simulink model "Arm_Mobile_Simulation_MATLAB24"  (R2024b)
settings: Solver=ode23t  StartTime=0.0  StopTime=25  MaxStep=dt  RelTol=1e-3
InitFcn:
  | dt = 0.01;
  | 
  | OP = 1;
  | 
  | %% Contact Data
  | G_K = 1e6;
  | G_B = 1e3;
  | 
  | G_Mu_s = 0.3;
  | G_Mu_k = 0.5;
  | 
  | %% Object Position for Pick and Drop
  | 
  | PL = [1.2 0 0.675];  % Pick location
  | 
  | PD = [1.4 0.8 0.475]; % Drop location
  | 
  | 
  | %% SimData
  | % Simscape(TM) Multibody(TM) version: 7.4
  | 
  | % This is a model data file derived from a Simscape Multibody Import XML file using the smimport function.
  | % The data in this file sets the block parameter values in an imported Simscape Multibody model.
  | % For more information on this file, see the smimport function help page in the Simscape Multibody documentation.
  | % You can modify numerical values, but avoid any other changes to this file.
  | % Do not add code to this file. Do not edit the physical units shown in comments.
  | 
  | %%%VariableName:smiData
  | 
  | 
  | %============= RigidTransform =============%
  | 
  | 
  | %Initialize the RigidTransform structure array by filling in null values.
  | smiData.RigidTransform(13).translation = [0.0 0.0 0.0];
  | smiData.RigidTransform(13).angle = 0.0;
  | smiData.RigidTransform(13).axis = [0.0 0.0 0.0];
  | smiData.RigidTransform(13).ID = '';
  | 
  | %Translation Method - Cartesian
  | %Rotation Method - Arbitrary Axis
  | smiData.RigidTransform(1).translation = [112.76762317970824 466.03898900587342 544.6225551646221];  % mm
  | smiData.RigidTransform(1).angle = 2.0943951023931953;  % rad
  | smiData.RigidTransform(1).axis = [-0.57735026918962584 -0.57735026918962584 -0.57735026918962584];
  | smiData.RigidTransform(1).ID = 'B[J1-1:-:J2-1]';
  | 
  | %Translation Method - Cartesian
  | %Rotation Method - Arbitrary Axis
  | smiData.RigidTransform(2).translation = [112.76762317970881 466.03898900587347 544.62255516462187];  % mm
  | smiData.RigidTransform(2).angle = 2.0943951023931957;  % rad
  | smiData.RigidTransform(2).axis = [-0.57735026918962584 -0.57735026918962573 -0.57735026918962573];
  | smiData.RigidTransform(2).ID = 'F[J1-1:-:J2-1]';
  | 
  | %Translation Method - Cartesian
  | %Rotation Method - Arbitrary Axis
  | smiData.RigidTransform(3).translation = [122.68366911264206 748.03898900587353 274.20311793228069];  % mm
  | smiData.RigidTransform(3).angle = 2.2406646857653398;  % rad
  | smiData.RigidTransform(3).axis = [0.61891214827171492 0.61891214827171503 0.48362744488229914];
  | smiData.RigidTransform(3).ID = 'B[J2-1:-:J3-1]';
  | 
  | ... (+181 lines)
undefined symbols (not defined in the file): smiData, X, Y, Z
libraries: sm_lib x161, nesl_utility x26
(part 4 of 4)

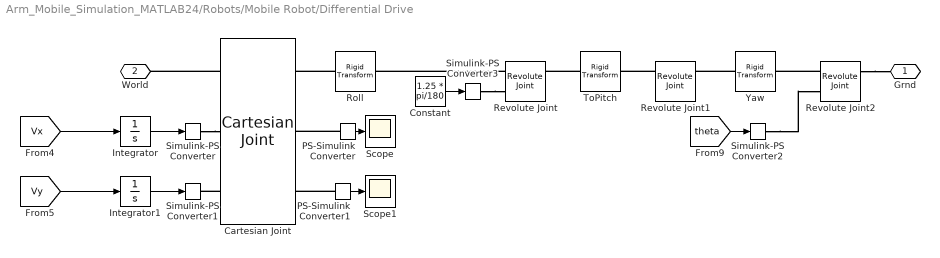
== system Arm_Mobile_Simulation_MATLAB24/Robots/Mobile Robot/Differential Drive ==
  Cartesian Joint : sm_lib/Joints/Cartesian Joint  JointMode=Normal  CompositeWrenchDir=FollowerOnBase  CompositeWrenchFrame=BaseFrame  SenseConstraintForce=off  SenseConstraintTorque=off  SenseTotalForce=off  SenseTotalTorque=off  PxPositionTargetSpecify=off  PxPositionTargetPriority=High  PxPositionTargetValue=0  PxPositionTargetValueUnits=m  PxVelocityTargetSpecify=off  PxVelocityTargetPriority=High  PxVelocityTargetValue=0  PxVelocityTargetValueUnits=m/s  PxEquilibriumPosition=0  PxEquilibriumPositionUnits=m  PxSpringStiffness=0  PxSpringStiffnessUnits=N/m  PxDampingCoefficient=0  PxDampingCoefficientUnits=N/(m/s)  PxLowerLimitSpecify=off  PxLowerLimitBound=-1  PxLowerLimitBoundUnits=m  PxLowerLimitStiffness=1e6  PxLowerLimitStiffnessUnits=N/m  PxLowerLimitDamping=1e3  PxLowerLimitDampingUnits=N/(m/s)  PxLowerLimitTransitionRegionWidth=1e-4  PxLowerLimitTransitionRegionWidthUnits=m  PxUpperLimitSpecify=off  PxUpperLimitBound=1  PxUpperLimitBoundUnits=m  PxUpperLimitStiffness=1e6  PxUpperLimitStiffnessUnits=N/m  PxUpperLimitDamping=1e3  PxUpperLimitDampingUnits=N/(m/s)  PxUpperLimitTransitionRegionWidth=1e-4  PxUpperLimitTransitionRegionWidthUnits=m  PxTorqueActuationMode=ComputedTorque  PxMotionActuationMode=InputMotion  PxSensePosition=on  PxSenseVelocity=off  PxSenseAcceleration=off  PxSenseTorqueForce=off  PxSenseLowerLimitTorqueForce=off  PxSenseUpperLimitTorqueForce=off  PyPositionTargetSpecify=off  PyPositionTargetPriority=High  PyPositionTargetValue=0  PyPositionTargetValueUnits=m  PyVelocityTargetSpecify=off  PyVelocityTargetPriority=High  PyVelocityTargetValue=0  PyVelocityTargetValueUnits=m/s  PyEquilibriumPosition=0  PyEquilibriumPositionUnits=m  PySpringStiffness=0  PySpringStiffnessUnits=N/m  PyDampingCoefficient=0  PyDampingCoefficientUnits=N/(m/s)  PyLowerLimitSpecify=off  PyLowerLimitBound=-1  PyLowerLimitBoundUnits=m  PyLowerLimitStiffness=1e6  PyLowerLimitStiffnessUnits=N/m  PyLowerLimitDamping=1e3  PyLowerLimitDampingUnits=N/(m/s)  PyLowerLimitTransitionRegionWidth=1e-4  PyLowerLimitTransitionRegionWidthUnits=m  PyUpperLimitSpecify=off  PyUpperLimitBound=1  PyUpperLimitBoundUnits=m  PyUpperLimitStiffness=1e6  PyUpperLimitStiffnessUnits=N/m  PyUpperLimitDamping=1e3  PyUpperLimitDampingUnits=N/(m/s)  PyUpperLimitTransitionRegionWidth=1e-4  PyUpperLimitTransitionRegionWidthUnits=m  PyTorqueActuationMode=ComputedTorque  PyMotionActuationMode=InputMotion  PySensePosition=on  PySenseVelocity=off  PySenseAcceleration=off  PySenseTorqueForce=off  PySenseLowerLimitTorqueForce=off  PySenseUpperLimitTorqueForce=off  PzPositionTargetSpecify=off  PzPositionTargetPriority=High  PzPositionTargetValue=0  PzPositionTargetValueUnits=m  PzVelocityTargetSpecify=off  PzVelocityTargetPriority=High  PzVelocityTargetValue=0  PzVelocityTargetValueUnits=m/s  PzEquilibriumPosition=0  PzEquilibriumPositionUnits=m  PzSpringStiffness=0  PzSpringStiffnessUnits=N/m  PzDampingCoefficient=0  PzDampingCoefficientUnits=N/(m/s)  PzLowerLimitSpecify=off  PzLowerLimitBound=-1  PzLowerLimitBoundUnits=m  PzLowerLimitStiffness=1e6  PzLowerLimitStiffnessUnits=N/m  PzLowerLimitDamping=1e3  PzLowerLimitDampingUnits=N/(m/s)  PzLowerLimitTransitionRegionWidth=1e-4  PzLowerLimitTransitionRegionWidthUnits=m  PzUpperLimitSpecify=off  PzUpperLimitBound=1  PzUpperLimitBoundUnits=m  PzUpperLimitStiffness=1e6  PzUpperLimitStiffnessUnits=N/m  PzUpperLimitDamping=1e3  PzUpperLimitDampingUnits=N/(m/s)  PzUpperLimitTransitionRegionWidth=1e-4  PzUpperLimitTransitionRegionWidthUnits=m  PzTorqueActuationMode=NoTorque  PzMotionActuationMode=ComputedMotion  PzSensePosition=off  PzSenseVelocity=off  PzSenseAcceleration=off  PzSenseTorqueForce=off  PzSenseLowerLimitTorqueForce=off  PzSenseUpperLimitTorqueForce=off
  Constant : Constant  Value=1.25 * pi/180
  Integrator : Integrator
  Integrator1 : Integrator
  PS-Simulink Converter : nesl_utility/PS-Simulink Converter  PhysicalDomain=network_engine_domain  SubClassName=ps_output  LeftPortType=input  RightPortType=output  PseudoPeriodic=off  Frequencies=[]  VectorFormat=1-D array  Unit=inherit  AffineConversion=off
  PS-Simulink Converter1 : nesl_utility/PS-Simulink Converter  PhysicalDomain=network_engine_domain  SubClassName=ps_output  LeftPortType=input  RightPortType=output  PseudoPeriodic=off  Frequencies=[]  VectorFormat=1-D array  Unit=inherit  AffineConversion=off
  Revolute Joint : sm_lib/Joints/Revolute Joint  JointMode=Normal  CompositeWrenchDir=FollowerOnBase  CompositeWrenchFrame=BaseFrame  SenseConstraintForce=off  SenseConstraintTorque=off  SenseTotalForce=off  SenseTotalTorque=off  PositionTargetSpecify=off  PositionTargetPriority=High  PositionTargetValue=90  PositionTargetValueUnits=deg  VelocityTargetSpecify=off  VelocityTargetPriority=High  VelocityTargetValue=0  VelocityTargetValueUnits=deg/s  EquilibriumPosition=0  EquilibriumPositionUnits=deg  SpringStiffness=0  SpringStiffnessUnits=N*m/deg  DampingCoefficient=0  DampingCoefficientUnits=N*m/(deg/s)  LowerLimitSpecify=off  LowerLimitBound=-90  LowerLimitBoundUnits=deg  LowerLimitStiffness=1e4  LowerLimitStiffnessUnits=N*m/deg  LowerLimitDamping=10  LowerLimitDampingUnits=N*m/(deg/s)  LowerLimitTransitionRegionWidth=0.1  LowerLimitTransitionRegionWidthUnits=deg  UpperLimitSpecify=off  UpperLimitBound=90  UpperLimitBoundUnits=deg  UpperLimitStiffness=1e4  UpperLimitStiffnessUnits=N*m/deg  UpperLimitDamping=10  UpperLimitDampingUnits=N*m/(deg/s)  UpperLimitTransitionRegionWidth=0.1  UpperLimitTransitionRegionWidthUnits=deg  TorqueActuationMode=ComputedTorque  MotionActuationMode=InputMotion  SensePosition=on  SenseVelocity=off  SenseAcceleration=off  SenseTorqueForce=off  SenseLowerLimitTorqueForce=off  SenseUpperLimitTorqueForce=off
  Revolute Joint1 : sm_lib/Joints/Revolute Joint  JointMode=Normal  CompositeWrenchDir=FollowerOnBase  CompositeWrenchFrame=BaseFrame  SenseConstraintForce=off  SenseConstraintTorque=off  SenseTotalForce=off  SenseTotalTorque=off  PositionTargetSpecify=off  PositionTargetPriority=High  PositionTargetValue=0.0234  PositionTargetValueUnits=rad  VelocityTargetSpecify=off  VelocityTargetPriority=High  VelocityTargetValue=0  VelocityTargetValueUnits=deg/s  EquilibriumPosition=0  EquilibriumPositionUnits=deg  SpringStiffness=0  SpringStiffnessUnits=N*m/deg  DampingCoefficient=0  DampingCoefficientUnits=N*m/(deg/s)  LowerLimitSpecify=off  LowerLimitBound=-90  LowerLimitBoundUnits=deg  LowerLimitStiffness=1e4  LowerLimitStiffnessUnits=N*m/deg  LowerLimitDamping=10  LowerLimitDampingUnits=N*m/(deg/s)  LowerLimitTransitionRegionWidth=0.1  LowerLimitTransitionRegionWidthUnits=deg  UpperLimitSpecify=off  UpperLimitBound=90  UpperLimitBoundUnits=deg  UpperLimitStiffness=1e4  UpperLimitStiffnessUnits=N*m/deg  UpperLimitDamping=10  UpperLimitDampingUnits=N*m/(deg/s)  UpperLimitTransitionRegionWidth=0.1  UpperLimitTransitionRegionWidthUnits=deg  TorqueActuationMode=ComputedTorque  MotionActuationMode=InputMotion  SensePosition=on  SenseVelocity=off  SenseAcceleration=off  SenseTorqueForce=off  SenseLowerLimitTorqueForce=off  SenseUpperLimitTorqueForce=off
  Revolute Joint2 : sm_lib/Joints/Revolute Joint  JointMode=Normal  CompositeWrenchDir=FollowerOnBase  CompositeWrenchFrame=BaseFrame  SenseConstraintForce=off  SenseConstraintTorque=off  SenseTotalForce=off  SenseTotalTorque=off  PositionTargetSpecify=off  PositionTargetPriority=High  PositionTargetValue=90  PositionTargetValueUnits=deg  VelocityTargetSpecify=off  VelocityTargetPriority=High  VelocityTargetValue=0  VelocityTargetValueUnits=deg/s  EquilibriumPosition=0  EquilibriumPositionUnits=deg  SpringStiffness=0  SpringStiffnessUnits=N*m/deg  DampingCoefficient=0  DampingCoefficientUnits=N*m/(deg/s)  LowerLimitSpecify=off  LowerLimitBound=-90  LowerLimitBoundUnits=deg  LowerLimitStiffness=1e4  LowerLimitStiffnessUnits=N*m/deg  LowerLimitDamping=10  LowerLimitDampingUnits=N*m/(deg/s)  LowerLimitTransitionRegionWidth=0.1  LowerLimitTransitionRegionWidthUnits=deg  UpperLimitSpecify=off  UpperLimitBound=90  UpperLimitBoundUnits=deg  UpperLimitStiffness=1e4  UpperLimitStiffnessUnits=N*m/deg  UpperLimitDamping=10  UpperLimitDampingUnits=N*m/(deg/s)  UpperLimitTransitionRegionWidth=0.1  UpperLimitTransitionRegionWidthUnits=deg  TorqueActuationMode=ComputedTorque  MotionActuationMode=InputMotion  SensePosition=on  SenseVelocity=off  SenseAcceleration=off  SenseTorqueForce=off  SenseLowerLimitTorqueForce=off  SenseUpperLimitTorqueForce=off
  Roll : sm_lib/Frames and Transforms/Rigid Transform  RotationMethod=AlignedAxes  FollAlignAxisA=+Z  BaseAlignAxisA=-X  FollAlignAxisB=+X  BaseAlignAxisB=+Y  RotationStandardAxis=+X  RotationAngle=90  RotationAngleUnits=deg  RotationArbitraryAxis=[0 0 1]  RotationSequenceAxes=FollowerAxes  RotationSequence=XYX  RotationSequenceAngles=[0 0 0]  RotationSequenceAnglesUnits=deg  RotationMatrix=[1 0 0; 0 1 0; 0 0 1]  Quaternion=[1 0 0 0]  TranslationMethod=None  TranslationCartesianOffset=[0 0 0]  TranslationCartesianOffsetUnits=m  TranslationStandardAxis=+Z  TranslationStandardOffset=0  TranslationStandardOffsetUnits=m  TranslationROffset=0  TranslationROffsetUnits=m  TranslationThetaOffset=0  TranslationThetaOffsetUnits=deg  TranslationZOffset=0  TranslationZOffsetUnits=m
  Scope : Scope
  Scope1 : Scope
  Simulink-PS Converter{,1..3} (4 alike) : nesl_utility/Simulink-PS Converter  PhysicalDomain=network_engine_domain  SubClassName=ps_input  LeftPortType=input  RightPortType=output  PseudoPeriodic=off  Frequencies=[]  NoiseDistribution=none  NoiseParameters=[]  Unit=1  AffineConversion=off  FilteringAndDerivatives=filter  SimscapeFilterOrder=2  InputFilterTimeConstant=0.001  UdotUserProvided=0
  ToPitch : sm_lib/Frames and Transforms/Rigid Transform  RotationMethod=StandardAxis  FollAlignAxisA=+X  BaseAlignAxisA=+Y  FollAlignAxisB=+Y  BaseAlignAxisB=+Z  RotationStandardAxis=-X  RotationAngle=90  RotationAngleUnits=deg  RotationArbitraryAxis=[0 0 1]  RotationSequenceAxes=FollowerAxes  RotationSequence=XYX  RotationSequenceAngles=[0 0 0]  RotationSequenceAnglesUnits=deg  RotationMatrix=[1 0 0; 0 1 0; 0 0 1]  Quaternion=[1 0 0 0]  TranslationMethod=None  TranslationCartesianOffset=[0 0 0]  TranslationCartesianOffsetUnits=m  TranslationStandardAxis=+Z  TranslationStandardOffset=0  TranslationStandardOffsetUnits=m  TranslationROffset=0  TranslationROffsetUnits=m  TranslationThetaOffset=0  TranslationThetaOffsetUnits=deg  TranslationZOffset=0  TranslationZOffsetUnits=m
  Yaw : sm_lib/Frames and Transforms/Rigid Transform  RotationMethod=StandardAxis  FollAlignAxisA=+X  BaseAlignAxisA=+Y  FollAlignAxisB=+Y  BaseAlignAxisB=+Z  RotationStandardAxis=+Y  RotationAngle=90  RotationAngleUnits=deg  RotationArbitraryAxis=[0 0 1]  RotationSequenceAxes=FollowerAxes  RotationSequence=XYX  RotationSequenceAngles=[0 0 0]  RotationSequenceAnglesUnits=deg  RotationMatrix=[1 0 0; 0 1 0; 0 0 1]  Quaternion=[1 0 0 0]  TranslationMethod=None  TranslationCartesianOffset=[0 0 0]  TranslationCartesianOffsetUnits=m  TranslationStandardAxis=+Z  TranslationStandardOffset=0  TranslationStandardOffsetUnits=m  TranslationROffset=0  TranslationROffsetUnits=m  TranslationThetaOffset=0  TranslationThetaOffsetUnits=deg  TranslationZOffset=0  TranslationZOffsetUnits=m
  Grnd : PMIOPort  Side=Right
  World : PMIOPort  Port=2  Side=Left
  wires:
  Integrator1/1 -> Simulink-PS Converter1/1
  Integrator/1 -> Simulink-PS Converter/1
  PS-Simulink Converter/1 -> Scope/1
  PS-Simulink Converter1/1 -> Scope1/1
  [Vy] -> Integrator1/1
  [Vx] -> Integrator/1
  Constant/1 -> Simulink-PS Converter3/1
  [theta] -> Simulink-PS Converter2/1
  connections:
  Revolute Joint2/LConn1 -- Yaw/LConn1
  Roll/RConn1 -- Cartesian Joint/RConn1
  ToPitch/RConn1 -- Revolute Joint/RConn1
  Yaw/RConn1 -- Revolute Joint1/RConn1
  Revolute Joint/LConn1 -- Roll/LConn1
  Revolute Joint1/LConn1 -- ToPitch/LConn1
  Cartesian Joint/LConn1 -- World/RConn1
  Revolute Joint2/RConn1 -- Grnd/RConn1
  Simulink-PS Converter/RConn1 -- Cartesian Joint/LConn2
  Cartesian Joint/LConn3 -- Simulink-PS Converter1/RConn1
  PS-Simulink Converter/LConn1 -- Cartesian Joint/RConn2
  PS-Simulink Converter1/LConn1 -- Cartesian Joint/RConn3
  Simulink-PS Converter2/RConn1 -- Revolute Joint2/LConn2
  Simulink-PS Converter3/RConn1 -- Revolute Joint/LConn2

== matlab function Arm_Mobile_Simulation_MATLAB24/Kinematics ==
  data: Vr input; w output; Vl input; V output
function [w, V] = fcn(Vr, Vl)

d = .162;

w = (Vr - Vl) / (2*d);


V = (Vr + Vl)/2;

== matlab function Arm_Mobile_Simulation_MATLAB24/for Robot ARm ==
  data: PL input; Theta output; PD input; r output; dt input
function [Theta, r] = fcn(PL, PD, dt)

% PL is the pickup location
% PD is the drop location

EEF_Rot_Des = [0 0 1; 0 -1 0; 1 0 0];% Orientation to grab the object from side. This depends upon the designer. One must analyze the kinematics to know how to get it

 % Tranformation matrix for pickup
T_PL = zeros(4,4);

T_PL([1 2 3],[1 2 3]) = EEF_Rot_Des;
T_PL([1 2 3],4) = [PL(1);PL(2);PL(3)+0.02];
T_PL(4,4) = 1;

 % Tranformation matrix for drop
T_PD = zeros(4,4);
T_PD([1 2 3],[1 2 3]) = EEF_Rot_Des;
T_PD([1 2 3],4) = [PD(1);PD(2);PD(3)+0.04];
T_PD(4,4) = 1;

% This function is just to maintain the variable from previous sampling time loop
% SO we don't have to output and then input to the function again

persistent ramp i GP
if isempty(ramp)

    % When the simulation starts, these must be the initial values.
    ramp = 0; % Ramp is just aan increment that will change the EEF trajectory
    i    = 2; % i is the 
    GP   = 0; % This is the command for gripper to hold or drop

end

Ini_T = [-1 0 0 0.26; 0 -1 0 0; 0 0 1 2.215; 0 0 0 1]; % Initial position of the robot

T_V1 = [-1 0 0 0.5; 0 -1 0 0; 0 0 1 1.8; 0 0 0 1]; % Via point for trajectory between initial position and picking. From here orientation will change

% Via point for trajectory between picking and dropping
T_V2 = zeros(4,4);

T_V2([1 2 3],[1 2 3]) = EEF_Rot_Des;
T_V2([1 2 3],4) = [PD(1);PD(2);PD(3)] - [0.1;0.3;-0.3];
T_V2(4,4) = 1;

% Via point for trajectory between dropping and initial
T_V3 = zeros(4,4);

T_V3([1 2 3],[1 2 3]) = EEF_Rot_Des;
T_V3([1 2 3],4) = [PD(1);PD(2);PD(3)] - [0.1;0;-0.1];
T_V3(4,4) = 1;

% FInal Trajectory Points
T_P = [Ini_T;T_V1;T_PL;T_V2;T_PD; T_V3; Ini_T];

% Speed

v = 0.5; % m/sec

% Making trajectory

T = Ini_T; % Initially, the trajectory is equal to the starting point of the robot

if i < 8 % Now the total movement of the robot between initial to picking and droping is composed of 4 points 

    Diff = T_P([-3:0]+4*i,:) - T_P([-3:0]+ (4*(i-1)),:); % This is just the difference between the current and the next moving point. 

    ramp = dt*v + ramp; % A ramp is generated from 0 to 1 so that the difference in previous step is generated and added to current point to reach the desired point

    if i == 4 && GP < 1 % So when the robot has reached the picking position, now it should grab the object before moving towards final point

        GP = 0.005 + GP; % So same like ramp, the gripper is gripping the object

        if GP >= 1 % This GP is bewteen 0 and 1

            GP = 1; % if it exceeds 1, then 1

        end

        if GP < 1 % While gripping, the ramp should remain 0

            ramp = ramp - dt*v; % SO the 0.005 added to the ramo in line 38 is compensated here again

        end

    end

    % Dropping

    if i == 6 && GP > 0 % So when the robot has reached the picking position, now it should grab the object before moving towards final point

        GP = -0.005 + GP; % So same like ramp, the gripper is gripping the object

        if GP <= 0 % This GP is bewteen 0 and 1

            GP = 0; % if it exceeds 1, then 1

        end

        if GP > 0 % While gripping, the ramp should remain 0

            ramp = ramp - dt*v; % SO the 0.005 added to the ramo in line 38 is compensated here again

        end

    end

    T = T_P([-3:0]+ (4*(i-1)),:) + Diff * ramp; % This is the trajectory for the EEF

    if ramp >= 1 % Now, onece the ramp reached 1, this means that one trajectory is completed

        ramp = 0; % Therefore, we have to reset the ramp to start new trajectory

        i = i+1; % And increment i by 1 so the next point is selected

    end


end

if i > 7 % if i > 7, thats mean the robot has reached all the 7 points

    T = T_P([-3:0]+ (4*(i-1)),:); % Now the trajectory is same as the last point

end

TD = T;

%% Inverse Kinematics
R06 = TD([1 2 3],[1 2 3]);
P06 = TD([1 2 3],4);

% These are the lenghs of the robot
L1 = .675;
L2 = .260;
L3 = .680;
L4 = .470;
L5 = .190;
L6 = .158;
L7 = .042;

% Inverse Kinematics Equations
L = L6 + L7;

Pc = P06 - L* R06([1 2 3],3); 

Xc = Pc(1);
Yc = Pc(2);
Zc = Pc(3);

% Theta 1
t1 = atan2(Yc,Xc);

% Theta 3
% r = sqrt((Xc - L2*cos(t1))^2 + (Yc - L2*sin(t1))^2);

r = sqrt((Xc)^2 + (Yc)^2) - L2;
s = Zc - L1;

c3 = (r^2 + s^2 - L3^2 - (L4+L5)^2) / (2*L3*(L4+L5));
s3 = real(sqrt(1 - c3^2));

t3 = atan2(s3,c3) - 1.5708;

% Theta 2

k1 = L3 + (L4+L5)*c3;
k2 = (L4+L5)*s3;

t2 = -atan2(s,r) - atan2(k2,k1);

% DH Table
d1=L1        ; a1=L2        ;  alpha1 = -90;
d2=0         ; a2=L3        ;  alpha2 =  00;
d3=0         ; a3=0         ;  alpha3 = -90;
d4=L4+L5     ; a4=0         ;  alpha4 = 90;
d5=0         ; a5=0         ;  alpha5 = -90;
d6=L6+L7     ; a6=0         ;  alpha6 =  0;

% Transformation
A1 =  [cos(t1) -sin(t1)*cosd(alpha1) sin(t1)*sind(alpha1) a1*cos(t1);
       sin(t1) cos(t1)*cosd(alpha1)  -cos(t1)*sind(alpha1) a1*sin(t1);
       0            sind(alpha1)            cosd(alpha1)         d1;
       0                0                 0                1];
   
A2 =  [cos(t2) -sin(t2)*cosd(alpha2) sin(t2)*sind(alpha2) a2*cos(t2);
       sin(t2) cos(t2)*cosd(alpha2)  -cos(t2)*sind(alpha2) a2*sin(t2);
       0            sind(alpha2)            cosd(alpha2)         d2;
       0                0                 0                1];
A3 =  [cos(t3) -sin(t3)*cosd(alpha3) sin(t3)*sind(alpha3) a3*cos(t3);
       sin(t3) cos(t3)*cosd(alpha3)  -cos(t3)*sind(alpha3) a3*sin(t3);
       0            sind(alpha3)            cosd(alpha3)         d3;
       0                0                 0                1];

% First three joint
T03 = A1*A2*A3;
R03 = T03([1 2 3],[1 2 3]);

R03i = inv(R03); % Inverse of R03

R36n = R03i * R06; % Calculated R36

% Theta 5
c5 = R36n(3,3);
s5 = sqrt(1 - c5^2);

t5 = atan2(s5,c5);

if P06(2) == 0 || R06(1,3) ~= 0

    t5 = -t5;

end

% Theta 4
c4 = -R36n(1,3)/(-s5);

if R06(3,3) < 0

    c4 = -R36n(1,3)/(s5);

end

if abs(c4) > 1
    
    c4 = sign(c4)*1;

end


s4 = real(sqrt(1 - c4^2));
t4 = atan2(s4,c4);

if P06(2) == 0

    t4 = 0;

end

% Theta 6
s6 = R36n(3,2)/(s5);
c6 = sqrt(1 - s6^2);
t6 = atan(s6/c6);

%% Output
Theta = [t1 t2 t3 t4 t5 t6];

r = 0.016 * GP; % r is the gripper position. 0.006 is multipled because the each finger of gripper should move only 5mm. Here 1 extra mm is for perfect gripping

== matlab function Arm_Mobile_Simulation_MATLAB24/Inv Kinecmatics ==
  data: v input; vx output; t input; vy output
function [vx,vy] = fcn(v,t)

vx = v*sin(-t);
vy = v*cos(-t);

== matlab function Arm_Mobile_Simulation_MATLAB24/MATLAB Function1 ==
  settings: updateMethod=DISCRETE
  data: CF input; Vr output; Vl output; dt input
function [Vr, Vl] = fcn(CF, dt)

% Global variable which needs to be maintained without initializing them
% everytime.
persistent clk Contact
if isempty(clk)

    clk     = 0;
    Contact = 0;

end

Vr = 0; % Right wheel m/sec
Vl = 0; % Left wheel m/sec

% First It detect the contact
if CF == 1 && Contact == 0

    Contact = 1;

end

if Contact == 1

    if clk > 1

        % Forward Movement
        if clk <= 4
    
            Vr = 1;
            Vl = 1;
    
        end
    
        % Turn Right 180 Degree
        if clk > 4 && clk <= 6
    
            Vr = 0.5;
            Vl = 1;
    
        end
    
        % Turn left 180 Degree
        if clk > 6 && clk <= 8
    
            Vr = 1;
            Vl = 0.5;
    
        end

        % Go Forward
        if clk > 8 && clk <= 8.5
    
            Vr = 1;
            Vl = 1;
    
        end

    end

    % Timer clock for mobile robot
    clk = clk + dt;

end
